simulink model "ej0214_modeloSimu"  (R2023a)
settings: Solver=VariableStepAuto  StartTime=0.0  StopTime=10.0  RelTol=1e-3
values from neighbouring files (symbols this model uses):
  As = [0,1;-1/L/C,-R/L]    [ej0214_simulink.m]
  Bs = [0;1/L/C]    [ej0214_simulink.m]
  C = 6e-3    (= 0.006)    [ej0214_simulink.m]
  Cs = [1 0;0 C;-1 -R*C;0 R*C]    [ej0214_simulink.m]
  Ds = [0;0;1;0]    [ej0214_simulink.m]
  L = 3    [ej0214_simulink.m]
  R = 250    [ej0214_simulink.m]
settings Model: Creator=cjuar  LastModifiedBy=cjuar

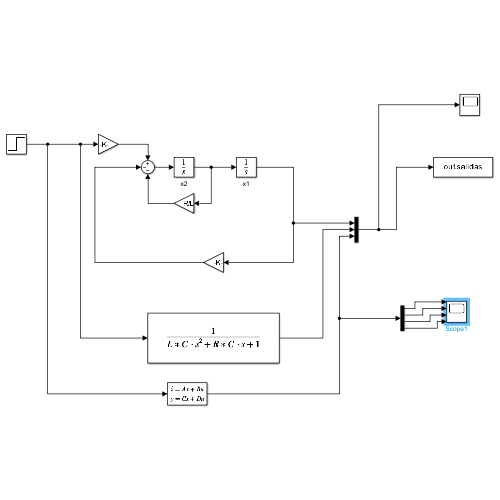
[thumbnail: Simulink's stored preview of the top-level diagram]
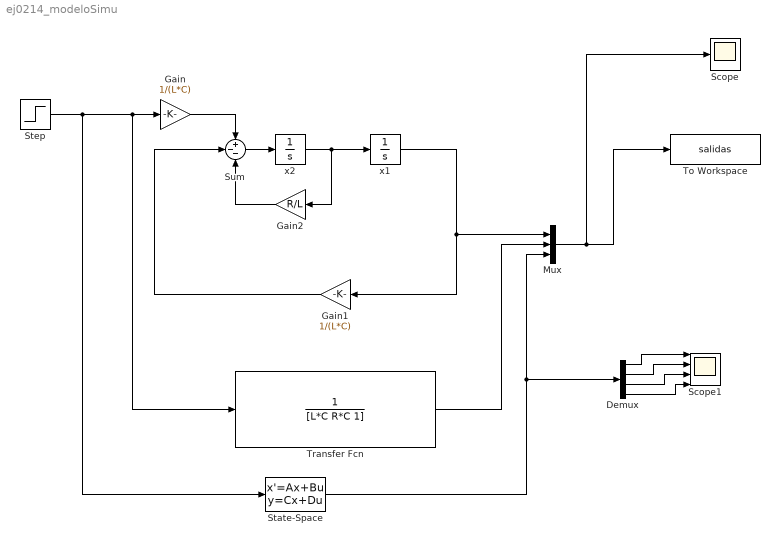
== system ej0214_modeloSimu ==
  Demux : Demux
  Gain : Gain  Gain=1/(L*C)
  Gain1 : Gain  Gain=1/(L*C)
  Gain2 : Gain  Gain=R/L
  Mux : Mux  Inputs=3
  Scope : Scope
  Scope1 : Scope  NumInputPorts=4
  State-Space : StateSpace  A=As  B=Bs  C=Cs  D=Ds  InitialCondition=0
  Step : Step  SampleTime=0
  Sum : Sum  Inputs=+--
  To Workspace : ToWorkspace  VariableName=salidas  SaveFormat=Timeseries  SampleTime=-1
  Transfer Fcn : TransferFcn  Denominator=[L*C R*C 1]
  x1 : Integrator
  x2 : Integrator
  wires:
  x2/1 -> Gain2/1, x1/1
  x1/1 -> Mux/1, Gain1/1
  Step/1 -> State-Space/1, Transfer Fcn/1, Gain/1
  Gain/1 -> Sum/1
  Sum/1 -> x2/1
  Gain1/1 -> Sum/2
  Gain2/1 -> Sum/3
  Mux/1 -> Scope/1, To Workspace/1
  Transfer Fcn/1 -> Mux/2
  State-Space/1 -> Mux/3, Demux/1
  Demux/1 -> Scope1/1
  Demux/2 -> Scope1/2
  Demux/3 -> Scope1/3
  Demux/4 -> Scope1/4
